simulink library "libCmdPowConversion"  (R2020b)
settings: Solver=VariableStepAuto  StartTime=0.0  StopTime=10.0  RelTol=1e-3
settings Model: Creator=caatay  LastModifiedBy=caatay

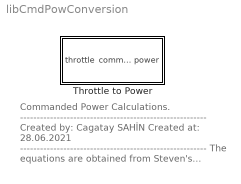
== system libCmdPowConversion ==
  note: Commanded Power Calculations.
      | --------------------------------------------------------
      | Created by: Cagatay SAHİN
      | Created at: 28.06.2021
      | --------------------------------------------------------
      | The equations are obtained from
      | Steven's textbook.
      | The reference book can be found in
      | "references folder".
      | --------------------------------------------------------
      | for question:
      | cagataysahin44@gmail.com
  Throttle to Power : Subsystem  mask(Engine Model - Throttle Command to Power Conversion){}
      mask help: Aircraft's commanded power calculation/conversion with using throttle command.
      mask Help:
      | This block is used for obtain commanded power with using commanded throttle.
      | --------------------------------------------------------------------------------------------------------------------------------------------------
      | Input of the function:
      | 	throttle: Throttle Command.
      | Output of the function:
      | 	cmdPow: Commanded Power
      | --------------------------------------------------------------------------------------------------------------------------------------------------
      | All equations can be found in Steven's text book. Reference can be found in "literature" subfolder.
      | for question: "cagataysahin44@gmail.com"
      mask Display:
      | port_label('input',1,'\delta_{t}','texmode','on');
      | 
      | port_label('output',1,'Pow_{cmd}','texmode','on');

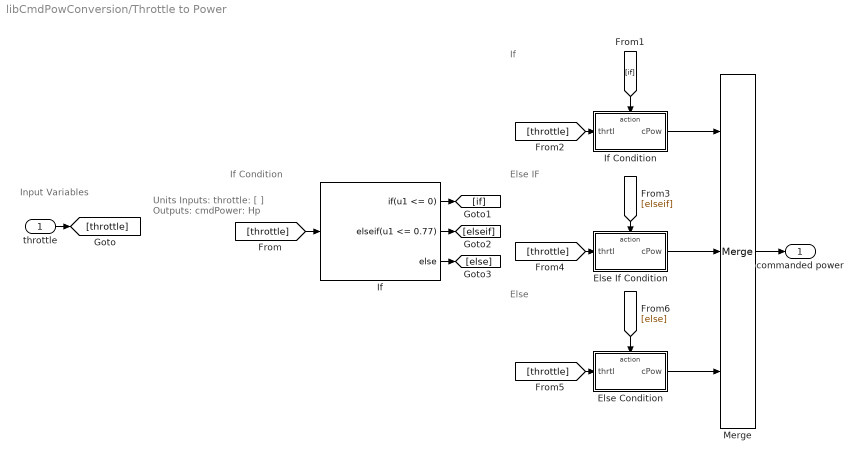
== system libCmdPowConversion/Throttle to Power ==
  note: If
  note: Else
  note: Input Variables
  note: Else IF
  note: If Condition
  note: Units
      | Inputs:
      | throttle: [ ]
      | Outputs:
      | cmdPower: Hp
  throttle : Inport
  Else Condition : Subsystem  TreatAsAtomicUnit=on
  Else If Condition : Subsystem  TreatAsAtomicUnit=on
  If : If  IfExpression=u1 <= 0  ElseIfExpressions=u1 <= 0.77
  If Condition : Subsystem  TreatAsAtomicUnit=on
  Merge : Merge  Inputs=3
  commanded power : Outport  VectorParamsAs1DForOutWhenUnconnected=off
  wires:
  [else] -> Else Condition/Action
  Else Condition/1(cPow) -> Merge/3
  [elseif] -> Else If Condition/Action
  [throttle] -> Else Condition/1(thrtl)
  Merge/1 -> commanded power/1
  If Condition/1(cPow) -> Merge/1
  throttle/1 -> [throttle]
  If/2 -> [elseif]
  [throttle] -> If/1
  [throttle] -> If Condition/1(thrtl)
  [if] -> If Condition/Action
  If/3 -> [else]
  If/1 -> [if]
  Else If Condition/1(cPow) -> Merge/2
  [throttle] -> Else If Condition/1(thrtl)

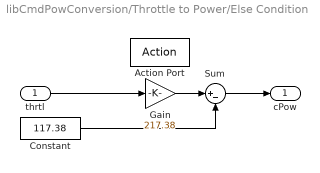
== system libCmdPowConversion/Throttle to Power/Else Condition ==
  thrtl : Inport
  Action Port : ActionPort
  Constant : Constant  Value=117.38
  Gain : Gain  Gain=217.38
  Sum : Sum  Inputs=|+-
  cPow : Outport  VectorParamsAs1DForOutWhenUnconnected=off
  wires:
  thrtl/1 -> Gain/1
  Gain/1 -> Sum/1
  Constant/1 -> Sum/2
  Sum/1 -> cPow/1

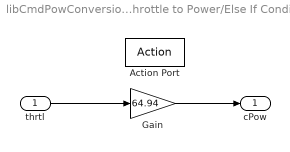
== system libCmdPowConversion/Throttle to Power/Else If Condition ==
  thrtl : Inport
  Action Port : ActionPort
  Gain : Gain  Gain=64.94
  cPow : Outport  VectorParamsAs1DForOutWhenUnconnected=off
  wires:
  thrtl/1 -> Gain/1
  Gain/1 -> cPow/1

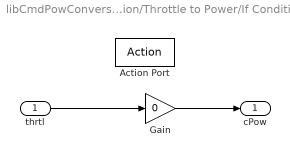
== system libCmdPowConversion/Throttle to Power/If Condition ==
  thrtl : Inport
  Action Port : ActionPort
  Gain : Gain  Gain=0
  cPow : Outport  VectorParamsAs1DForOutWhenUnconnected=off
  wires:
  thrtl/1 -> Gain/1
  Gain/1 -> cPow/1
